simulink model "ArduCopter_MinnieLindiCopter"  (R2018b)
settings: Solver=FixedStepDiscrete  StartTime=0.0  StopTime=1000  FixedStep=lindiCopter_params.ts  RelTol=1e-4
libraries: ardupilot_custom_controller_lib x2, simulink x1, lindiCopter_lib x1, axes_transformation_lib x1
settings Model: DataTypeOverride=Single  DataTypeOverrideAppliesTo=Floating-point  Creator=Yannic  LastModifiedBy=yannic
settings SolverCC: ZeroCrossControl=DisableAll
settings DataIOCC: LimitDataPoints=on  SaveOutput=off  SaveTime=off  ReturnWorkspaceOutputs=on
settings OptimizationCC: DefaultParameterBehavior=Inlined  UseFloatMulNetSlope=on  DefaultUnderspecifiedDataType=single  InlineInvariantSignals=on  PassReuseOutputArgsAs=Individual arguments  ZeroExternalMemoryAtStartup=off  ZeroInternalMemoryAtStartup=off  NoFixptDivByZeroProtection=on  EfficientFloat2IntCast=on  LifeSpan=1  OptimizeBlockOrder=speed  DifferentSizesBufferReuse=on
settings DebuggingCC: ReadBeforeWriteMsg=DisableAll  WriteAfterWriteMsg=DisableAll  WriteAfterReadMsg=DisableAll  MultiTaskDSMMsg=none  ParameterPrecisionLossMsg=none  ParameterTunabilityLossMsg=error  AllowSymbolicDim=off  LibraryContextMissingDiagnostic=none  SFUnexpectedBacktrackingDiag=warning  SFNoUnconditionalDefaultTransitionDiag=warning  SFExecutionAtInitializationDiag=none  UnderSpecifiedDimensionMsg=warning
settings HardwareCC: ProdBitPerPointer=32  ProdBitPerSizeT=32  ProdBitPerPtrDiffT=32  ProdLargestAtomicInteger=Long  ProdWordSize=32  ProdHWDeviceType=ARM Compatible->ARM 7
settings ModelReferenceCC: UpdateModelReferenceTargets=IfOutOfDate  PropagateSignalLabelsOutOfModel=off
settings SFSimCC: SFSimEcho=off  SimUseLocalCustomCode=off  MATLABDynamicMemAlloc=off
settings RTWCC: SystemTargetFile=ert.tlc  GenCodeOnly=on  TemplateMakefile=ert_default_tmf  GenerateReport=on  RTWUseLocalCustomCode=off  IncludeHyperlinkInReport=on  LaunchReport=on  TargetLang=C++  GenerateTraceInfo=on  GenerateTraceReport=on  GenerateTraceReportSl=on  GenerateTraceReportSf=on  GenerateTraceReportEml=on
settings CodeAppCC: ForceParamTrailComments=on  IgnoreCustomStorageClasses=off  OperatorAnnotations=on  SimulinkDataObjDesc=on  SFDataObjDesc=on  CustomSymbolStrGlobalVar=rt$N$M  CustomSymbolStrType=$N$M  CustomSymbolStrFcn=$N$M$F  CustomSymbolStrMacro=$N$M  InsertBlockDesc=on
settings ERTTargetCC: TargetLangStandard=C++03 (ISO)  GenerateSampleERTMain=on  IncludeMdlTerminateFcn=off  CombineSignalStateStructs=on  SuppressErrorStatus=on  SupportAbsoluteTime=off  MultiInstanceERTCode=on  CodeInterfacePackaging=C++ class  SupportNonFinite=off  SupportVariableSizeSignals=on  ERTHeaderFileRootName=MatlabController$E  ERTSourceFileRootName=MatlabController$E  ERTDataFileRootName=MatlabController_data  InlinedParameterPlacement=NonHierarchical  RootIOFormat=Structure reference  ERTCustomFileTemplate=example_file_process.tlc  ERTFilePackagingFormat=CompactWithDataFile
settings ConfigComp: CovMetricSettings=dw  CovHtmlReporting=on  CovSaveCumulativeToWorkspaceVar=on  CovSaveSingleToWorkspaceVar=on  CovExternalEMLEnable=off

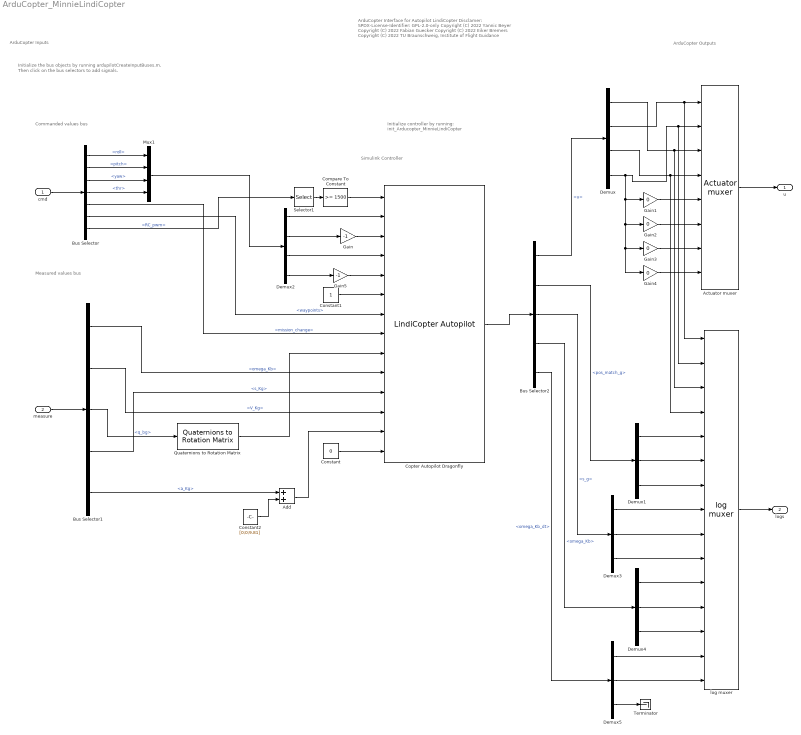
== system ArduCopter_MinnieLindiCopter ==
  note: Measured values bus
  note: Initialize the bus objects by running ardupilotCreateInputBuses.m.
      | Then click on the bus selectors to add signals.
  note: Commanded values bus
  note: ArduCopter Inputs
  note: ArduCopter Outputs
  note: Simulink Controller
  note: Initialize controller by running:
      | init_Arducopter_MinnieLindiCopter
  note: ArduCopter Interface for Autopilot LindiCopter
      |
      | Disclamer:
      | SPDX-License-Identifier: GPL-2.0-only
      |
      | Copyright (C) 2022 Yannic Beyer
      | Copyright (C) 2022 Fabian Guecker
      | Copyright (C) 2022 Eiker Bremers
      | Copyright (C) 2022 TU Braunschweig, Institute of Flight Guidance
  cmd : Inport  OutDataTypeStr=Bus: cmdBus
  measure : Inport  Port=2  OutDataTypeStr=Bus: measureBus
  Actuator muxer : ardupilot_custom_controller_lib/Actuator muxer
      settings: SourceProductName=LADAC
  Add : Sum
  Bus Selector : BusSelector  OutputSignals=roll,pitch,yaw,thr,mission_change,waypoints,RC_pwm
  Bus Selector1 : BusSelector  OutputSignals=omega_Kb,V_Kg,q_bg,s_Kg,a_Kg
  Bus Selector2 : BusSelector  OutputSignals=inner_loop_indi.u,guidance.matching.pos_match_g,pos_cntrl.measure.s_g,atti_cntrl.measure.omega_Kb,atti_cntrl.measure.omega_Kb_dt
  Compare To Constant : simulink/Logic and Bit Operations/Compare To Constant  relop=>=  const=1500  OutDataTypeStr=uint8
  Constant : Constant  Value=0
  Constant1 : Constant
  Constant2 : Constant  Value=[0;0;9.81]  OutDataTypeStr=Inherit: Inherit via back propagation
  Copter Autopilot Dragonfly : lindiCopter_lib/LindiCopter Autopilot  ap=lindiCopter_params
  Demux : Demux
  Demux{1,3..5} (4 alike) : Demux  Outputs=3
  Demux2 : Demux
  Gain : Gain  Gain=-1
  Gain{1..4} (4 alike) : Gain  Gain=0
  Gain5 : Gain  Gain=-1
  Mux1 : Mux
  Quaternions to Rotation Matrix : axes_transformation_lib/Quaternions to Rotation Matrix  SystemSampleTime=-1
      settings: SourceProductName=LADAC
  Selector1 : Selector  InputPortWidth=16  IndexOptions=Index vector (dialog)  Indices=7  OutputSizes=1
  Terminator : Terminator
  log muxer : ardupilot_custom_controller_lib/log muxer  batch_name_1='ML1'  num_signals_1=14  batch_name_2='ML2'  num_signals_2=1  batch_name_3='ML3'  num_signals_3=0  batch_name_4='ML4'  num_signals_4=0  batch_name_5='ML5'  num_signals_5=0
      settings: SourceProductName=LADAC
  u : Outport
  logs : Outport  Port=2
  wires:
  cmd/1 -> Bus Selector/1
  measure/1 -> Bus Selector1/1
  Bus Selector/1 -> Mux1/1  "<roll>"
  Bus Selector/2 -> Mux1/2  "<pitch>"
  Bus Selector/3 -> Mux1/3  "<yaw>"
  Bus Selector/4 -> Mux1/4  "<thr>"
  Actuator muxer/1 -> u/1
  log muxer/1 -> logs/1
  Gain1/1 -> Actuator muxer/5
  Demux/2 -> log muxer/1, Actuator muxer/1
  Demux/4 -> log muxer/2, Actuator muxer/2, Gain1/1, Gain4/1, Gain3/1, Gain2/1
  Demux/1 -> log muxer/3, Actuator muxer/3
  Demux/3 -> log muxer/4, Actuator muxer/4
  Demux1/1 -> log muxer/5
  Demux1/2 -> log muxer/6
  Demux1/3 -> log muxer/7
  Demux3/1 -> log muxer/8
  Demux3/2 -> log muxer/9
  Demux3/3 -> log muxer/10
  Demux4/1 -> log muxer/11
  Demux4/2 -> log muxer/12
  Demux5/1 -> log muxer/14
  Demux5/2 -> log muxer/15
  Gain/1 -> Copter Autopilot Dragonfly/3
  Quaternions to Rotation Matrix/1 -> Copter Autopilot Dragonfly/9
  Bus Selector1/2 -> Copter Autopilot Dragonfly/12  "<V_Kg>"
  Demux2/4 -> Gain5/1
  Mux1/1 -> Demux2/1
  Bus Selector1/1 -> Copter Autopilot Dragonfly/10  "<omega_Kb>"
  Demux2/2 -> Gain/1
  Demux2/3 -> Copter Autopilot Dragonfly/4
  Bus Selector1/4 -> Copter Autopilot Dragonfly/11  "<s_Kg>"
  Constant/1 -> Copter Autopilot Dragonfly/14
  Demux2/1 -> Copter Autopilot Dragonfly/2
  Bus Selector1/3 -> Quaternions to Rotation Matrix/1  "<q_bg>"
  Copter Autopilot Dragonfly/1 -> Bus Selector2/1
  Bus Selector2/1 -> Demux/1  "<u>"
  Gain2/1 -> Actuator muxer/6
  Gain3/1 -> Actuator muxer/7
  Gain4/1 -> Actuator muxer/8
  Bus Selector/5 -> Copter Autopilot Dragonfly/8  "<mission_change>"
  Bus Selector/6 -> Copter Autopilot Dragonfly/7  "<waypoints>"
  Bus Selector/7 -> Selector1/1  "<RC_pwm>"
  Compare To Constant/1 -> Copter Autopilot Dragonfly/1
  Selector1/1 -> Compare To Constant/1
  Bus Selector2/2 -> Demux1/1  "<pos_match_g>"
  Bus Selector2/3 -> Demux3/1  "<s_g>"
  Gain5/1 -> Copter Autopilot Dragonfly/5
  Constant1/1 -> Copter Autopilot Dragonfly/6
  Bus Selector2/4 -> Demux4/1  "<omega_Kb>"
  Demux4/3 -> log muxer/13
  Bus Selector2/5 -> Demux5/1  "<omega_Kb_dt>"
  Demux5/3 -> Terminator/1
  Bus Selector1/5 -> Add/1  "<a_Kg>"
  Add/1 -> Copter Autopilot Dragonfly/13
  Constant2/1 -> Add/2
